simulink model "Omnidirectional_robot_special_case_Lars_Method_R2019a"  (R2019a)
settings: Solver=FixedStepAuto  StartTime=0.0  StopTime=60.0  FixedStep=1e-2  RelTol=1e-3
libraries: simulink x1
settings Model: Creator=Admin  LastModifiedBy=Admin

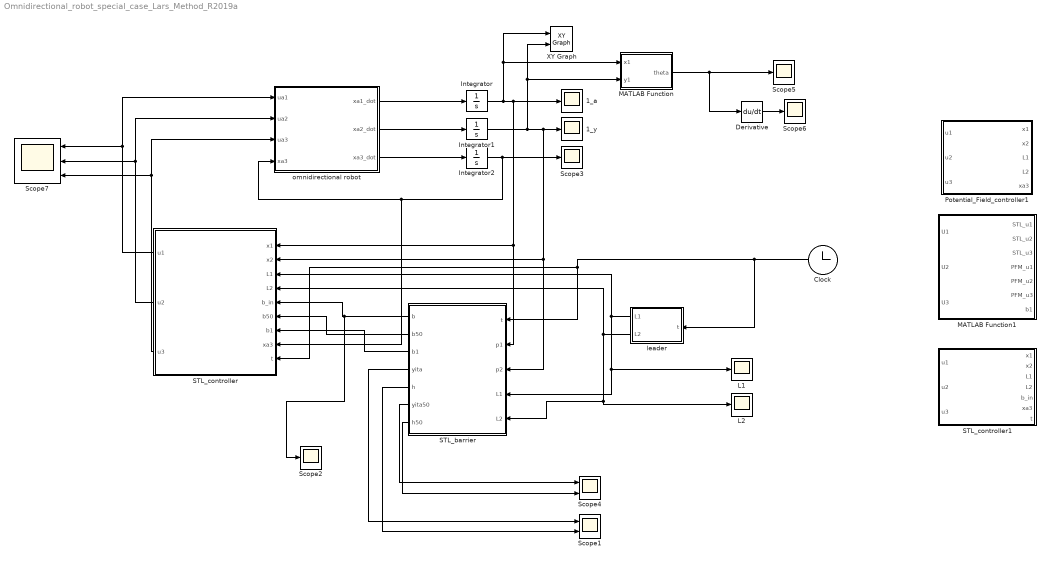
== system Omnidirectional_robot_special_case_Lars_Method_R2019a ==
  1_a : Scope
  1_y : Scope
  Clock : Clock
  Derivative : Derivative
  Integrator : Integrator
  Integrator1 : Integrator  InitialCondition=5
  Integrator2 : Integrator
  L1 : Scope
  L2 : Scope
  MATLAB Function : MATLAB Function  TreatAsAtomicUnit=on
  MATLAB Function1 : MATLAB Function  TreatAsAtomicUnit=on
  Potential_Field_controller1 : MATLAB Function  TreatAsAtomicUnit=on
  "STL_barrier " : MATLAB Function  TreatAsAtomicUnit=on
  STL_controller : MATLAB Function  TreatAsAtomicUnit=on
  STL_controller1 : MATLAB Function  TreatAsAtomicUnit=on
  Scope1 : Scope  NumInputPorts=2
  Scope{2..3,5..6} (4 alike) : Scope
  Scope4 : Scope  NumInputPorts=2
  Scope7 : Scope  NumInputPorts=3
  XY Graph : simulink/Sinks/XY Graph  xmin=-15  xmax=100  ymin=-15  ymax=100  st=0.01
  leader : MATLAB Function  TreatAsAtomicUnit=on
  omnidirectional robot : MATLAB Function  TreatAsAtomicUnit=on
  wires:
  omnidirectional robot/1(xa1_dot) -> Integrator/1
  Derivative/1 -> Scope6/1
  MATLAB Function/1(theta) -> Derivative/1, Scope5/1
  Integrator1/1 -> MATLAB Function/2(y1), XY Graph/2, "STL_barrier "/3(p2), STL_controller/2(x2), 1_y/1
  "STL_barrier "/4(yita) -> Scope1/1
  "STL_barrier "/5(h) -> Scope1/2
  Integrator2/1 -> omnidirectional robot/4(xa3), STL_controller/8(xa3), Scope3/1
  omnidirectional robot/3(xa3_dot) -> Integrator2/1
  Integrator/1 -> MATLAB Function/1(x1), XY Graph/1, "STL_barrier "/2(p1), STL_controller/1(x1), 1_a/1
  Clock/1 -> leader/1(t), STL_controller/9(t), "STL_barrier "/1(t)
  omnidirectional robot/2(xa2_dot) -> Integrator1/1
  leader/1(L1) -> L1/1, "STL_barrier "/4(L1), STL_controller/3(L1)
  leader/2(L2) -> L2/1, "STL_barrier "/5(L2), STL_controller/4(L2)
  "STL_barrier "/6(yita50) -> Scope4/1
  "STL_barrier "/7(h50) -> Scope4/2
  "STL_barrier "/1(b) -> Scope2/1, STL_controller/5(b_in)
  "STL_barrier "/2(b50) -> STL_controller/6(b50)
  "STL_barrier "/3(b1) -> STL_controller/7(b1)
  STL_controller/1(u1) -> Scope7/1, omnidirectional robot/1(ua1)
  STL_controller/2(u2) -> Scope7/2, omnidirectional robot/2(ua2)
  STL_controller/3(u3) -> Scope7/3, omnidirectional robot/3(ua3)

== matlab function Omnidirectional_robot_special_case_Lars_Method_R2019a/STL_barrier  ==
  data: b output; b50 output; b1 output; yita output; h output; t input; p1 input; p2 input; L1 input; L2 input; yita50 output; h50 output
function [b,b50,b1,yita,h,yita50,h50] = fcn(t,p1,p2,L1,L2)
d1=L1;
d2=L2;

d11=50;
d22=0;

b1=25*exp(-0.37*t)+7-sqrt( (p1-d1)^2 + (p2-d2)^2 );
yita=-25*exp(-0.37*t)+5;
h=12-sqrt( (p1-d1)^2 + (p2-d2)^2 );

b50=55*exp(-0.12*t)+5-sqrt( (p1-d11)^2 + (p2-d22)^2 );
yita50=-55*exp(-0.12*t)+5;
h50=10-sqrt( (p1-d11)^2 + (p2-d22)^2 );

% b50=5-sqrt( (p1-d11)^2 + (p2-d22)^2 );
% yita50=5;
% h50=10-sqrt( (p1-d11)^2 + (p2-d22)^2 );

%b1=sqrt( (p1-d11)^2 + (p2-d22)^2 )-4.2;
b=-(1/2)*log(exp(-2*b1)+exp(-2*b50));

== matlab function Omnidirectional_robot_special_case_Lars_Method_R2019a/omnidirectional robot ==
  data: ua1 input; xa1_dot output; ua2 input; ua3 input; xa3 input; xa2_dot output; xa3_dot output
function [xa1_dot,xa2_dot,xa3_dot]= fcn(ua1,ua2,ua3,xa3)

Li=0.2;
Bi=[0,cos(pi/6),-cos(pi/6);
    -1,sin(pi/6),sin(pi/6);
    Li,Li,Li;];

R1=[cos(xa3),-sin(xa3),0;
    sin(xa3),cos(xa3),0;
    0,0,1;];
R=0.02;

A=R1*inv(Bi')*R*[ua1;ua2;ua3];
xa1_dot=A(1,1);
xa2_dot=A(2,1);
xa3_dot=A(3,1);

== matlab function Omnidirectional_robot_special_case_Lars_Method_R2019a/STL_controller ==
  data: x1 input; x2 input; L1 input; L2 input; b_in input; b50 input; b1 input; u1 output; xa3 input; u2 output; u3 output; t input
function [u1,u2,u3]= fcn(x1, x2,L1,L2, b_in,b50,b1, xa3,t)
coder.extrinsic('quadoptimizer');
%coder.extrinsic('save');

d1=L1; d2=L2;
d11=50;d22=0;
partial_b_b1=(-1/2) * ( 1/( exp(-2*b1)+exp(-2*b50) ) ) * ( -2*exp(-2*b1) );
partial_b_b50=(-1/2) * ( 1/( exp(-2*b1)+exp(-2*b50) ) ) * ( -2*exp(-2*b50) );

partial_b1=(1/2)*((x1-d1)^2+(x2-d2)^2)^(-1/2);
partial_b1_x=[-2*partial_b1*partial_b_b1*(x1-d1),-2*partial_b1*partial_b_b1*(x2-d2),0];
partial_b50=(1/2)*((x1-d11)^2+(x2-d22)^2)^(-1/2);
partial_b50_x=[-2*partial_b50*partial_b_b50*(x1-d11),-2*partial_b50*partial_b_b50*(x2-d22),0];
partial_b_x=partial_b1_x+partial_b50_x;

Li=0.2;
Bi=[0,cos(pi/6),-cos(pi/6);
    -1,sin(pi/6),sin(pi/6);
    Li,Li,Li;];

R1=[cos(xa3),-sin(xa3),0;
    sin(xa3),cos(xa3),0;
    0,0,1;];
R=0.02;

gx=R1*inv(Bi')*R;

A=[partial_b_x*gx,1];

H=[0.1,0,0,0;
    0,0.1,0,0;
    0,0,0.1,0;
    0,0,0,0.9;];
%H=[1];
partial_b1_t=-0.37*25*exp(-0.37*t);
partial_b50_t=-0.12*55*exp(-0.12*t);
b=500*b_in+partial_b_b1*partial_b1_t+partial_b_b50*partial_b50_t+20;



u1=0;u2=0;u3=0;
U=quadoptimizer(H,b,A);

%U=quadprod(H,[],-A,b);

u1=U(1,1);
u2=U(2,1);
u3=U(3,1);

== matlab function Omnidirectional_robot_special_case_Lars_Method_R2019a/MATLAB Function ==
  data: x1 input; theta output; y1 input
function theta = fcn(x1, y1)
theta=atan2(y1,x1);

== matlab function Omnidirectional_robot_special_case_Lars_Method_R2019a/STL_controller1 ==
  data: x1 input; x2 input; L1 input; L2 input; b_in input; u1 output; xa3 input; u2 output; u3 output; t input
function [u1,u2,u3]= fcn(x1, x2,L1,L2, b_in, xa3,t)
coder.extrinsic('quadoptimizer');
%coder.extrinsic('save');
d1=50; d2=0;

partial_b=(1/2)*((x1-d1)^2+(x2-d2)^2)^(-1/2);
partial_b_x=[-2*partial_b*(x1-d1),-2*partial_b*(x2-d2),0];


Li=0.2;
Bi=[0,cos(pi/6),-cos(pi/6);
    -1,sin(pi/6),sin(pi/6);
    Li,Li,Li;];

R1=[cos(xa3),-sin(xa3),0;
    sin(xa3),cos(xa3),0;
    0,0,1;];
R=0.02;

gx=R1*inv(Bi')*R;

A=partial_b_x*gx;

H=[1,0,0;0,1,0;0,0,1];
%H=[1];

b=300*b_in-0.12*55*exp(-0.12*t)-50;
%  b=500*b_in-50;


u1=0;u2=0;u3=0;
U=quadoptimizer(H,b,A);

%U=quadprod(H,[],-A,b);

u1=U(1,1);
u2=U(2,1);
u3=U(3,1);

== matlab function Omnidirectional_robot_special_case_Lars_Method_R2019a/MATLAB Function1 ==
  data: STL_u1 input; U1 output; STL_u2 input; STL_u3 input; PFM_u1 input; PFM_u2 input; PFM_u3 input; b1 input; U2 output; U3 output
function [U1,U2,U3] = fcn(STL_u1,STL_u2,STL_u3,PFM_u1,PFM_u2,PFM_u3,b1)
U_goal=[STL_u1;STL_u2;STL_u3];
U_obs=[PFM_u1;PFM_u2;PFM_u3];
k=0.15;
lambda=1-exp(-k*max(b1,0));
U=lambda*U_goal+(1-lambda)*U_obs;
% U=U_goal;
U1=0;U2=0;U3=0;
U1=U(1,1);
U2=U(2,1);
U3=U(3,1);

== matlab function Omnidirectional_robot_special_case_Lars_Method_R2019a/leader ==
  data: t input; L1 output; L2 output
function [L1,L2] = fcn(t)
L1=30*sin(1*t);
L2=30*cos(1*t);

== matlab function Omnidirectional_robot_special_case_Lars_Method_R2019a/Potential_Field_controller1 ==
  data: x1 input; x2 input; L1 input; L2 input; u1 output; xa3 input; u2 output; u3 output
function [u1,u2,u3] = fcn(x1, x2,L1,L2, xa3)
coder.extrinsic('Calculate_gradient');
coder.extrinsic('PVF_optimizer');
coder.extrinsic('add_random');
A1=[-1,0;0,-1];
F=[2*L1,2*L2];
distance=sqrt((x1-90)^2+(x2-90)^2);
gradient_x=0;gradient_y=0;
[gradient_x,gradient_y]=Calculate_gradient(x1,x2,A1,F,50,50,20);
% gradient_x=Gradient(1,1);
% gradient_y=Gradient(1,2);
gradient_z=0;
Gradient_all=[gradient_x;gradient_y;gradient_z];

Li=0.2;
Bi=[0,cos(pi/6),-cos(pi/6);
    -1,sin(pi/6),sin(pi/6);
    Li,Li,Li;];

R1=[cos(xa3),-sin(xa3),0;
    sin(xa3),cos(xa3),0;
    0,0,1;];
R=0.02;
gx=R1*inv(Bi')*R;
A=Gradient_all'*gx;

%H=[1];
%H=[1,0;0,1];
%H=[0,0,0;0,0,0;0,0,0];
% H=[1,0,0;0,1,0;0,0,1];
 H=(1/2)*gx'*gx;
b=[0];
F=[-2*gx'*50*Gradient_all];
%=[];
u1=0;u2=0;u3=0;
U=PVF_optimizer(H,b,A,F,distance,gradient_x,gradient_y);

u1=U(1,1);
u2=U(2,1);
u3=U(3,1);
